simulink model "bai3"  (R2018b)
settings: Solver=FixedStepAuto  StartTime=0.0  StopTime=1  FixedStep=0.0001  RelTol=1e-3
undefined symbols (not defined in the file): J, KE, KT, La, OmegaN, Ra, Td, Tf, Zeta
settings Model: Creator=User  LastModifiedBy=User

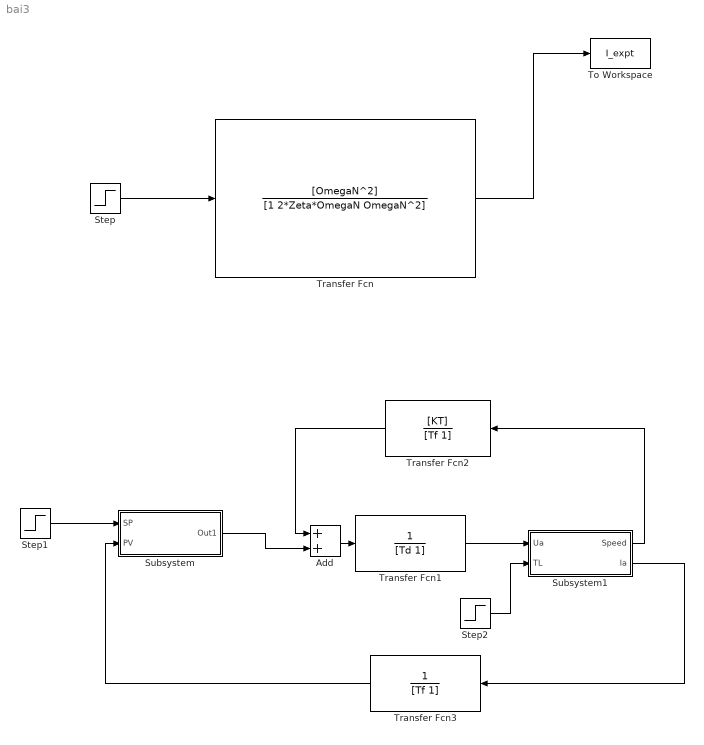
== system bai3 ==
  Add : Sum
  Step : Step  Time=0  After=62.5  SampleTime=0
  Step1 : Step  Time=0  After=62.5  SampleTime=0
  Step2 : Step  Time=0.5  After=70  SampleTime=0
  Subsystem : Subsystem
  Subsystem1 : Subsystem
  To Workspace : ToWorkspace  VariableName=I_expt  SaveFormat=Timeseries  SampleTime=-1
  Transfer Fcn : TransferFcn  Numerator=[OmegaN^2]  Denominator=[1 2*Zeta*OmegaN OmegaN^2]
  Transfer Fcn1 : TransferFcn  Denominator=[Td 1]
  Transfer Fcn2 : TransferFcn  Numerator=[KT]  Denominator=[Tf 1]
  Transfer Fcn3 : TransferFcn  Denominator=[Tf 1]
  wires:
  Step/1 -> Transfer Fcn/1
  Transfer Fcn/1 -> To Workspace/1
  Step1/1 -> Subsystem/1(SP)
  Transfer Fcn1/1 -> Subsystem1/1(Ua)
  Transfer Fcn3/1 -> Subsystem/2(PV)
  Subsystem1/2(Ia) -> Transfer Fcn3/1
  Step2/1 -> Subsystem1/2(TL)
  Add/1 -> Transfer Fcn1/1
  Subsystem/1(Out1) -> Add/2
  Subsystem1/1(Speed) -> Transfer Fcn2/1
  Transfer Fcn2/1 -> Add/1

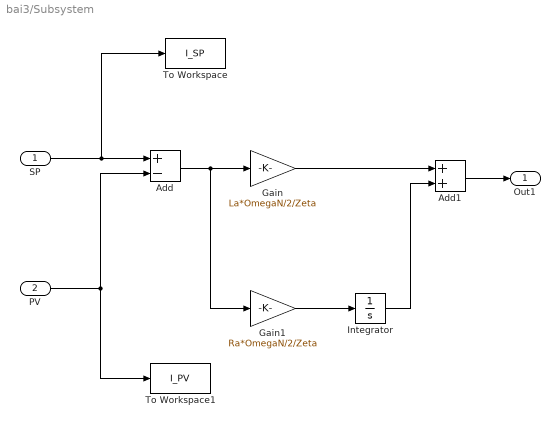
== system bai3/Subsystem ==
  SP : Inport
  PV : Inport  Port=2
  Add : Sum  Inputs=+-
  Add1 : Sum
  Gain : Gain  Gain=La*OmegaN/2/Zeta
  Gain1 : Gain  Gain=Ra*OmegaN/2/Zeta
  Integrator : Integrator
  To Workspace : ToWorkspace  VariableName=I_SP  SaveFormat=Timeseries  SampleTime=-1
  To Workspace1 : ToWorkspace  VariableName=I_PV  SaveFormat=Timeseries  SampleTime=-1
  Out1 : Outport
  wires:
  SP/1 -> To Workspace/1, Add/1
  PV/1 -> Add/2, To Workspace1/1
  Add/1 -> Gain1/1, Gain/1
  Gain1/1 -> Integrator/1
  Gain/1 -> Add1/1
  Integrator/1 -> Add1/2
  Add1/1 -> Out1/1

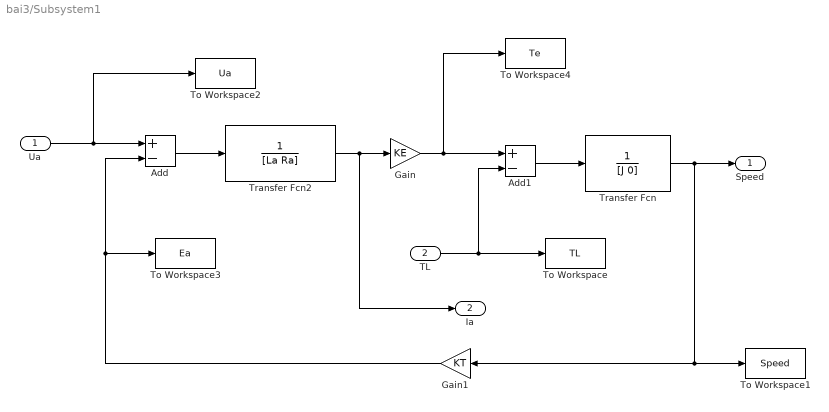
== system bai3/Subsystem1 ==
  Ua : Inport
  TL : Inport  Port=2
  Add : Sum  Inputs=+-
  Add1 : Sum  Inputs=+-
  Gain : Gain  Gain=KE
  Gain1 : Gain  Gain=KT
  To Workspace : ToWorkspace  VariableName=TL  SaveFormat=Timeseries  SampleTime=-1
  To Workspace1 : ToWorkspace  VariableName=Speed  SaveFormat=Timeseries  SampleTime=-1
  To Workspace2 : ToWorkspace  VariableName=Ua  SaveFormat=Timeseries  SampleTime=-1
  To Workspace3 : ToWorkspace  VariableName=Ea  SaveFormat=Timeseries  SampleTime=-1
  To Workspace4 : ToWorkspace  VariableName=Te  SaveFormat=Timeseries  SampleTime=-1
  Transfer Fcn : TransferFcn  Denominator=[J 0]
  Transfer Fcn2 : TransferFcn  Denominator=[La Ra]
  Speed : Outport
  Ia : Outport  Port=2
  wires:
  Add/1 -> Transfer Fcn2/1
  Transfer Fcn2/1 -> Ia/1, Gain/1
  Gain/1 -> To Workspace4/1, Add1/1
  Add1/1 -> Transfer Fcn/1
  Transfer Fcn/1 -> Gain1/1, To Workspace1/1, Speed/1
  TL/1 -> Add1/2, To Workspace/1
  Gain1/1 -> To Workspace3/1, Add/2
  Ua/1 -> To Workspace2/1, Add/1
